simulink model "LGVI_AS"  (R2017a)
settings: Solver=FixedStepDiscrete  StartTime=0.0  StopTime=10.0  RelTol=1e-3
settings Model: Creator=somup  LastModifiedBy=ssingh30

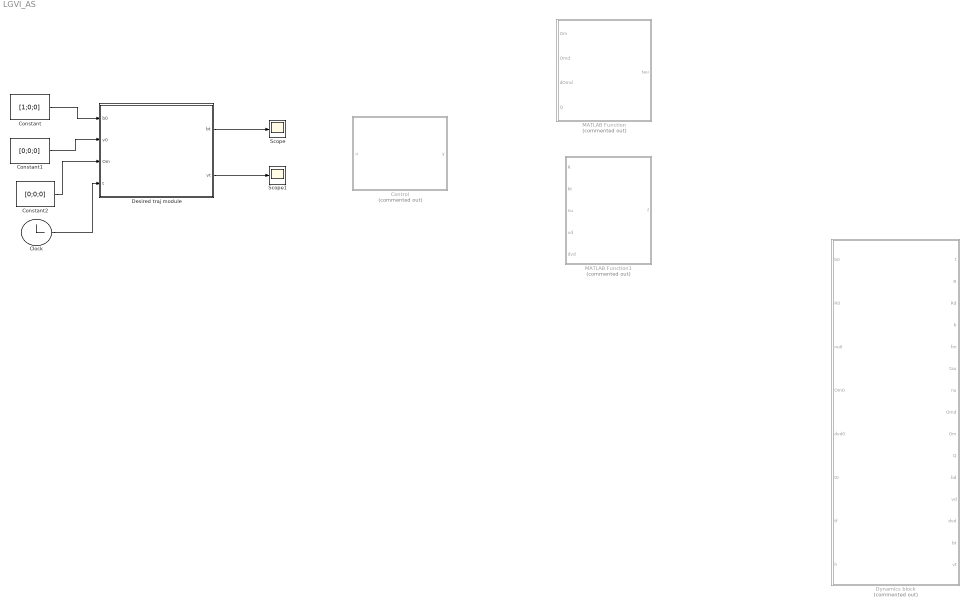
== system LGVI_AS ==
  Clock : Clock
  Constant : Constant  Value=[1;0;0]  VectorParams1D=off
  Constant1 : Constant  Value=[0;0;0]  VectorParams1D=off
  Constant2 : Constant  Value=[0;0;0]  VectorParams1D=off
  Control : MATLAB Function  Commented=on  TreatAsAtomicUnit=on
  Desired traj module : MATLAB Function  TreatAsAtomicUnit=on
  Dynamics block : MATLAB Function  Commented=on  TreatAsAtomicUnit=on
  MATLAB Function : MATLAB Function  Commented=on  TreatAsAtomicUnit=on
  MATLAB Function1 : MATLAB Function  Commented=on  TreatAsAtomicUnit=on
  Scope : Scope
  Scope1 : Scope
  wires:
  Constant1/1 -> Desired traj module/2(v0)
  Constant/1 -> Desired traj module/1(b0)
  Clock/1 -> Desired traj module/4(t)
  Desired traj module/1(bt) -> Scope/1
  Desired traj module/2(vt) -> Scope1/1
  Constant2/1 -> Desired traj module/3(Om)

== matlab function LGVI_AS/MATLAB Function ==
  data: Om input; tau output; Omd input; dOmd input; Q input
function tau =attitude_control_tau(Om,Omd,dOmd,Q)
global J p La ki kp e1 e2 e3
% parameter
L=La;
a1 = 1.2;
a2 = 1.1;
a3 = 1;

om=Om-Q'*Omd;

s = a1*cross(Q'*e1,e1)+a2*cross(Q'*e2,e2)+a3*cross(Q'*e3,e3);
H = eye(3,3)-((2*(1-(1/p)))/(s'*s))*(s*s');
w = a1*cross(e1,cross(om,Q'*e1))+a2*cross(e2,cross(om,Q'*e2))+a3*cross(e3,cross(om,Q'*e3));
z = s/((s'*s)^(1-(1/p)));
Psi = om+ki*z;




%dOmd=dOm+(ki/((s'*s)^(1-(1/p))))*H*w;

%tau=skew(Q'*Omd)*J*Om+J*(Q'*dOmd-skew(om)*Q'*Omd)-((L*om)/(om'*L*om)^(1-(1/p)));

tau =J*(Q'*dOmd-(ki*H/(s'*s)^(1-(1/p)))*w)...
     +skew(Q'*Omd)*J*(Q'*Omd-ki*z)+ki*J*(cross(z,(Q'*Omd)))...
     +cross(ki*J*(w+Q'*Omd),z)-kp*s...
     -(L*Psi/(Psi'*L*Psi)^(1-(1/p)));

== matlab function LGVI_AS/Control ==
  data: u input; y output
function y = fcn(u)

y = u;

== matlab function LGVI_AS/MATLAB Function1 ==
  data: R input; f output; bt input; nu input; vd input; dvd input
function f =trans_control_f(R,bt,nu,vd,dvd)

global L e3 g m P
% parameter

f = e3'*R'*(m*g*e3+P*bt+L*(R*nu-vd)-m*dvd);
%f=m*g*e3+P*bt+L*(R*nu-vd)-m*dvd;

== matlab function LGVI_AS/Dynamics block ==
  data: b0 input; t output; R0 input; nu0 input; Om0 input; dvd0 input; t0 input; tf input; h input; R output; Rd output; b output; fm output; tau output; nu output; Omd output; Om output; Q output; bd output; vd output; dvd output; bt output; vt output
function [t,R,Rd,b,fm,tau,nu,Omd,Om,Q,bd,vd,dvd,bt,vt] = LGVI_SE3_UAV(b0,R0,nu0,Om0,dvd0,t0,tf,h)

global J M m e3 g 
% UAV parameters 
J=diag([0.0820,0.0845,0.1377]);         % kgm^2; UAV inertia; 3 x 3 matrix
m=4.34;                                 % kg, mass of UAV
M=m*eye(3);                             % 
g=9.81;
e3=[0;0;1]'; 

b(:,1)=b0;
R(:,:,1)=R0;
nu(:,1)=[0;0;0];
Om(:,1)=[0;0;0];
Omd(:,1)=Om0;
%Rd(:,:,1)=R0;



Delt=tf-t0;                 % length of time interval; assumes tf > t0
n=fix(Delt/h);

t(1) = 0;
bd(:,1)=[0;0.6;0];
vd(:,1)=nu0;
dvd(:,1)=dvd0;


% t = linspace(t0,tf,tf/h);
t(1) = 0;
bd=[0.4*sin(pi*t);0.6*cos(pi*t);0.4*t];
vd=[0.4*pi*cos(pi*t);-0.6*pi*sin(pi*t);0.4*ones(size(t))];
dvd=[-0.4*pi^2*sin(pi*t);-0.6*pi^2*cos(pi*t); 0*ones(size(t))];

bt(:,1)=b0-bd(:,1);
vt(:,1)=R(:,:,1)*nu(:,1)-vd(:,1);
Rd(:,:,1)=desired_attitude(bt(:,1),vt(:,1),dvd(:,1));

%r1d(:,1)=[1;0;0];
for k=1:n-1
    t(k+1)=t(k)+h;
    k
    
%  bd(:,k+1)=[0.4*t(k+1);0.4*sin(pi*t(k+1));0.6*cos(pi*t(k+1))];
%  vd(:,k+1)=[0.4;0.4*pi*cos(pi*t(k+1));-0.6*pi*sin(pi*t(k+1))];
%  dvd(:,k+1)=[0;-0.4*pi^2*sin(pi*t(k+1));-0.6*pi^2*cos(pi*t(k+1))];
 
%  r1d(:,k+1)=[cos(pi*t(k+1));sin(pi*t(k+1));0];
%  bd=[0.4*t;0.4*sin(pi*t);0.6*cos(pi*t)] 
%  vd(:,k+1)=(1/h)*(bd(:,k+1)-bd(:,k));
%  dvd(:,k+1)=(1/h)*(vd(:,k+1)-vd(:,k));
%  vd=[0.4*ones(size(t));0.4*pi*cos(pi*t);-0.6*pi*sin(pi*t)];
 

%# Z motion waypoints   
bd(:,k+1)=[0.4*sin(pi*t(k+1));0.6*cos(pi*t(k+1));0.4*t(k+1)];
vd(:,k+1)=[0.4*pi*cos(pi*t(k+1));-0.6*pi*sin(pi*t(k+1));0.4];
dvd(:,k+1)=[-0.4*pi^2*sin(pi*t(k+1));-0.6*pi^2*cos(pi*t(k+1));0];

%dvd(:,k+1)=[0;0;0];
%      bd(:,k+1)=[0.4*sin(pi*t(k+1));0.6*cos(pi*t(k+1));0.4*t(k+1)];
%      vd(:,k+1)=[0.4*pi*cos(pi*t(k+1));-0.6*pi*sin(pi*t(k+1));0.4];
%      dvd(:,k+1)=[-0.4*pi^2*sin(pi*t(k+1));-0.6*pi^2*cos(pi*t(k+1));0];
    
   
%     bd(:,k)=[0.4*t;0.4*sin(pi*t);0.6*cos(pi*t)];
%     vd(:,k)=[0.4*ones(length(t));0.4*pi*cos(pi*t);-0.6*pi*sin(pi*t)];
%     dvd(:,k)=[zeros(length(t));-0.4*pi^2*sin(pi*t);-0.6*pi^2*cos(pi*t)]; 
 
%%%%%%%%%%%%%%%%%%%%%%%%%%%%%%%%%%%%% 
   % Solving the implicit equation of the kinematic eq's
    fi=h*Om(:,k);
%     nf=norm(fi);
%     G=sin(nf)/nf*J*fi+(1-cos(nf))/nf^2*cross(fi,J*fi);
%     while norm(G-h*J*Om(:,k)) > 1e-15
%         nf=norm(fi);
%         G=sin(nf)/nf*J*fi+(1-cos(nf))/nf^2*cross(fi,J*fi);
%         nabG=(cos(nf)*nf-sin(nf))/nf^3*(J*fi)*fi'+sin(nf)/nf*J...
%             +(sin(nf)*nf-2*(1-cos(nf)))/nf^4*cross(fi,J*fi)*fi'...
%             +(1-cos(nf))/nf^2*(skew(-J*fi)+[cross(fi,J(:,1)),cross(fi,J(:,2)),cross(fi,J(:,3))]);
%         fi=fi+inv(nabG)*(h*J*Om(:,k)-G);
%     end
    F(:,:,k)=expmso3(fi);
    %%%%%%%%%%%%%%%%%%%%%%%%%%%%%%%%%%%%%%
    
    R(:,:,k+1)=R(:,:,k)*F(:,:,k);       % next attitude
    b(:,k+1)=h*R(:,:,k)*nu(:,k)+b(:,k); % the next position
    
    % The control torque:
    bt(:,k+1)=b(:,k+1)-bd(:,k+1);
    fm(k)=trans_control_f(R(:,:,k),bt(:,k),nu(:,k),vd(:,k),dvd(:,k));
    
    nu(:,k+1)=M\(F(:,:,k)'*M*nu(:,k)+h*m*g*R(:,:,k+1)'*e3-h*fm(k)*e3);
   

    v(:,k+1)=R(:,:,k+1)*nu(:,k+1);
    vt(:,k+1)=v(:,k+1)-vd(:,k+1);
    
    Rd(:,:,k+1)=desired_attitude(bt(:,k+1),vt(:,k+1),dvd(:,k+1));
    
    Fd(:,:,k+1)=Rd(:,:,k)'*Rd(:,:,k+1);
    
    Omd(:,k+1)=(1/h)*(logmso3(Fd(:,:,k+1)));
    
    dOmd(:,k)=(1/h)*(Omd(:,k+1)-Omd(:,k));
    
    Q(:,:,k)=Rd(:,:,k)'*R(:,:,k);
    
    %om(:,k)=Om(:,k)-Q(:,:,k)'*Omd(:,k)
   
    tau(:,k)=attitude_control_tau(Om(:,k),Omd(:,k),dOmd(:,k),Q(:,:,k));
        
    Om(:,k+1)=J\((F(:,:,k)'*J*Om(:,k))+h*tau(:,k));
    
end

== matlab function LGVI_AS/Desired traj module ==
  data: b0 input; bt output; v0 input; Om input; t input; vt output
function [bt,vt] = des(b0,v0,Om,t)
J=diag([0.0820,0.0845,0.1377]);         % kgm^2; UAV inertia; 3 x 3 matrix
m=4.34;                                 % kg, mass of UAV
M=m*eye(3);                             % 
g=9.81;
e1=[1;0;0;];
e2=[0;1;0];
e3=[0;0;1];
% %initial inputs
% t(1)=0;
% b(:,1)=b0;
% v(:,1)=v0;
R0 = expSO3([0;0;0]);
% R0 = [1 0 0 ; 0 -1 0; 0 0 -1];
R = zeros(3);
R(:,:,1)= R0;


%desired trajectory function
t(1) = 0;
bd=[0.4*sin(pi*t);0.6*cos(pi*t);0.4*t];
vd=[0.4*pi*cos(pi*t);-0.6*pi*sin(pi*t);0.4];
dvd=[-0.4*pi^2*sin(pi*t);-0.6*pi^2*cos(pi*t); 0];

%now for n points to generate the trajectory
tf = 5;
t0=0;
h=0.01;
Delt=tf-t0;                 % length of time interval; assumes tf > t0
n=fix(Delt/h);

for k = 1:n-1
    t(k+1)=t(k)+h;
     
bd(:,k+1)=[0.4*sin(pi*t(k+1));0.6*cos(pi*t(k+1));0.4*t(k+1)];
vd(:,k+1)=[0.4*pi*cos(pi*t(k+1));-0.6*pi*sin(pi*t(k+1));0.4];
dvd(:,k+1)=[-0.4*pi^2*sin(pi*t(k+1));-0.6*pi^2*cos(pi*t(k+1));0];
%%%%%%%%%%%%%%%%%%%%%%%%%%%%%%%%%%%%% 
   % Solving the implicit equation of the kinematic eq's
    fi=h*Om(:,k);
%     nf=norm(fi);
%     G=sin(nf)/nf*J*fi+(1-cos(nf))/nf^2*cross(fi,J*fi);
%     while norm(G-h*J*Om(:,k)) > 1e-15
%         nf=norm(fi);
%         G=sin(nf)/nf*J*fi+(1-cos(nf))/nf^2*cross(fi,J*fi);
%         nabG=(cos(nf)*nf-sin(nf))/nf^3*(J*fi)*fi'+sin(nf)/nf*J...
%             +(sin(nf)*nf-2*(1-cos(nf)))/nf^4*cross(fi,J*fi)*fi'...
%             +(1-cos(nf))/nf^2*(skew(-J*fi)+[cross(fi,J(:,1)),cross(fi,J(:,2)),cross(fi,J(:,3))]);
%         fi=fi+inv(nabG)*(h*J*Om(:,k)-G);
%     end
    F = zeros(3);
    F(:,:,k)=expSO3(fi);

    R(:,:,k+1)=R(:,:,k)*F(:,:,k);       % next attitude
    b0(:,k+1)=h*R(:,:,k)*v0(:,k)+b0(:,k); % the next position
    
    % The control torque:
    bt(:,k+1)=b0(:,k+1)-bd(:,k+1);
 
    v0(:,k+1)=R(:,:,k+1)*v0(:,k+1);
    vt(:,k+1)=v0(:,k+1)-vd(:,k+1);

%calculation of error in traj
bt = b0 - bd ;
vt = v0 - vd ;
end
